simulink model "model20Drones"  (R2022a)
settings: Solver=FixedStepAuto  StartTime=0.0  StopTime=inf  FixedStep=1  RelTol=1e-3
values from neighbouring files (symbols this model uses):
  droneCount = 3    [workspace.mat]
  map = [0 0 0 0 0 0 0 0 0 0 99 99 ... (400 elements, 20x20)]    [workspace.mat]
libraries: drone x20
settings Model: Creator=JadKHaddad  LastModifiedBy=JadKHaddad

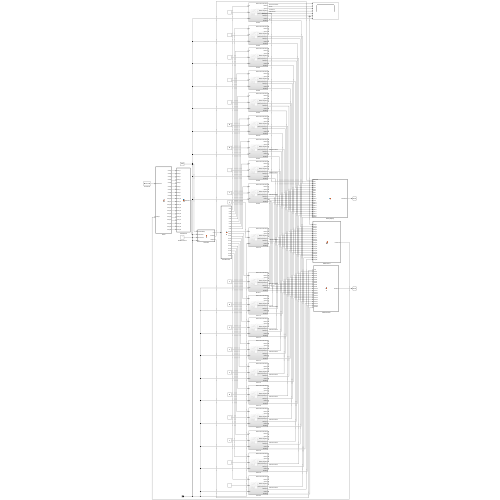
[thumbnail: Simulink's stored preview of the top-level diagram]
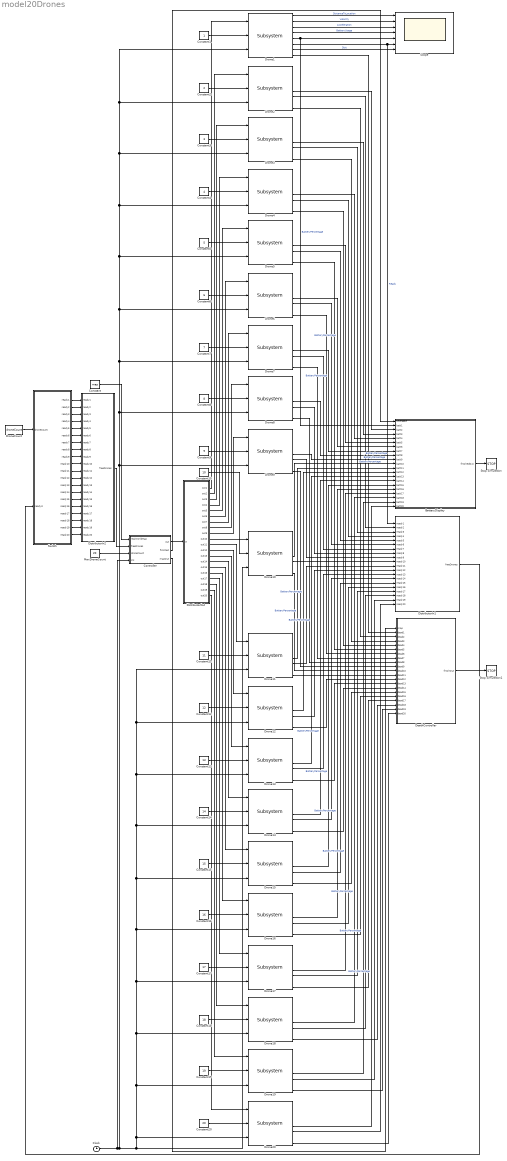
== system model20Drones ==
  BatteryDisplay : MATLAB Function  TreatAsAtomicUnit=on
  Clock : Clock
  Constant : Constant  Value=map  VectorParams1D=off
  Constant1 : Constant
  Constant10 : Constant  Value=10
  Constant11 : Constant  Value=11
  Constant12 : Constant  Value=12
  Constant13 : Constant  Value=13
  Constant14 : Constant  Value=14
  Constant15 : Constant  Value=15
  Constant16 : Constant  Value=16
  Constant17 : Constant  Value=17
  Constant18 : Constant  Value=18
  Constant19 : Constant  Value=19
  Constant2 : Constant  Value=2
  Constant20 : Constant  Value=20
  Constant3 : Constant  Value=3
  Constant4 : Constant  Value=4
  Constant5 : Constant  Value=5
  Constant6 : Constant  Value=6
  Constant7 : Constant  Value=7
  Constant8 : Constant  Value=8
  Constant9 : Constant  Value=9
  Controller : MATLAB Function  TreatAsAtomicUnit=on
  DeathController : MATLAB Function  TreatAsAtomicUnit=on
  DistributorIn1 : MATLAB Function  TreatAsAtomicUnit=on
  DistributorIn2 : MATLAB Function  TreatAsAtomicUnit=on
  DistributorOut : MATLAB Function  TreatAsAtomicUnit=on
  Drone{1..5,7..20} (19 alike) : drone/Subsystem  SystemSampleTime=-1  VariantActivationTime=update diagram  Latency=0  AutoFrameSizeCalculation=off
  "Drone6 " : drone/Subsystem  SystemSampleTime=-1  VariantActivationTime=update diagram  Latency=0  AutoFrameSizeCalculation=off
  DroneCount : Constant  Value=droneCount
  MaxDroneCount : Constant  Value=20
  Scope : Scope  NumInputPorts=7
  Stop Simulation : Stop
  Stop Simulation1 : Stop
  Switch : MATLAB Function  TreatAsAtomicUnit=on
  wires:
  Drone2/5 -> BatteryDisplay/3(batt2)
  DistributorOut/15(out15) -> Drone15/1
  Drone20/5 -> BatteryDisplay/21(batt20)  "BatteryPercentage"
  Switch/18(ready18) -> DistributorIn2/18(ready18)
  Drone19/5 -> BatteryDisplay/20(batt19)  "BatteryPercentage"
  Drone19/6 -> DistributorIn1/19(ready19)
  Constant13/1 -> Drone13/2
  Drone14/8 -> DeathController/15(dead14)
  DistributorOut/20(out20) -> Drone20/1
  Drone13/6 -> DistributorIn1/13(ready13)
  Clock/1 -> Drone12/3, Drone11/3, Drone13/3, Drone14/3, Drone15/3, Drone16/3, Drone17/3, Drone18/3, Drone19/3, Drone20/3, Drone10/3, Drone2/3, Drone1/3, Drone3/3, Drone4/3, Drone5/3, "Drone6 "/3, Drone7/3, Drone8/3, Drone9/3, Controller/4(clk)
  DistributorOut/19(out19) -> Drone19/1
  Drone17/8 -> DeathController/18(dead17)
  Drone20/6 -> DistributorIn1/20(ready20)
  Constant17/1 -> Drone17/2
  Switch/8(ready8) -> DistributorIn2/8(ready8)
  Drone19/8 -> DeathController/20(dead19)
  Drone11/5 -> BatteryDisplay/12(batt11)  "BatteryPercentage"
  Drone20/8 -> DeathController/21(dead20)
  Constant20/1 -> Drone20/2
  Switch/17(ready17) -> DistributorIn2/17(ready17)
  Drone15/5 -> BatteryDisplay/16(batt15)  "BatteryPercentage"
  Constant19/1 -> Drone19/2
  Drone18/5 -> BatteryDisplay/19(batt18)  "BatteryPercentage"
  Drone18/6 -> DistributorIn1/18(ready18)
  DistributorOut/5(out5) -> Drone5/1
  Drone18/8 -> DeathController/19(dead18)
  DistributorOut/18(out18) -> Drone18/1
  Drone11/6 -> DistributorIn1/11(ready11)
  Constant9/1 -> Drone9/2
  DistributorOut/17(out17) -> Drone17/1
  Constant18/1 -> Drone18/2
  Drone17/5 -> BatteryDisplay/18(batt17)  "BatteryPercentage"
  Drone17/6 -> DistributorIn1/17(ready17)
  Drone16/5 -> BatteryDisplay/17(batt16)  "BatteryPercentage"
  Drone16/8 -> DeathController/17(dead16)
  Drone16/6 -> DistributorIn1/16(ready16)
  Switch/12(ready12) -> DistributorIn2/12(ready12)
  DistributorOut/16(out16) -> Drone16/1
  Constant16/1 -> Drone16/2
  Drone15/6 -> DistributorIn1/15(ready15)
  Drone15/8 -> DeathController/16(dead15)
  Constant15/1 -> Drone15/2
  Switch/15(ready15) -> DistributorIn2/15(ready15)
  Drone14/6 -> DistributorIn1/14(ready14)
  Drone14/5 -> BatteryDisplay/15(batt14)  "BatteryPercentage"
  "Drone6 "/5 -> BatteryDisplay/7(batt6)  "BatteryPercentage"
  DistributorOut/14(out14) -> Drone14/1
  Constant14/1 -> Drone14/2
  Drone13/8 -> DeathController/14(dead13)
  Switch/5(ready5) -> DistributorIn2/5(ready5)
  Constant10/1 -> Drone10/2
  Switch/11(ready11) -> DistributorIn2/11(ready11)
  Switch/1(ready1) -> DistributorIn2/1(ready1)
  Drone13/5 -> BatteryDisplay/14(batt13)  "BatteryPercentage"
  DistributorOut/13(out13) -> Drone13/1
  Drone12/6 -> DistributorIn1/12(ready12)
  Drone12/8 -> DeathController/13(dead12)
  Drone12/5 -> BatteryDisplay/13(batt12)  "BatteryPercentage"
  DistributorOut/12(out12) -> Drone12/1
  Drone11/8 -> DeathController/12(dead11)
  Drone2/8 -> DeathController/3(dead2)
  Constant12/1 -> Drone12/2
  Constant11/1 -> Drone11/2
  DistributorOut/11(out11) -> Drone11/1
  Switch/20(ready20) -> DistributorIn2/20(ready20)
  Drone1/7 -> Scope/7  "Dist"
  Switch/19(ready19) -> DistributorIn2/19(ready19)
  Switch/16(ready16) -> DistributorIn2/16(ready16)
  Switch/14(ready14) -> DistributorIn2/14(ready14)
  Switch/13(ready13) -> DistributorIn2/13(ready13)
  Drone3/5 -> BatteryDisplay/4(batt3)
  Switch/4(ready4) -> DistributorIn2/4(ready4)
  Switch/3(ready3) -> DistributorIn2/3(ready3)
  DistributorOut/1(out1) -> Drone1/1
  DroneCount/1 -> Switch/1(droneCount)
  DistributorOut/3(out3) -> Drone3/1
  Drone2/6 -> DistributorIn1/2(ready2)
  Controller/2(finished) -> BatteryDisplay/1(finishedIn)
  DistributorOut/9(out9) -> Drone9/1
  Controller/3(mapOut) -> DeathController/1(map)
  DistributorIn2/1(freeDrones) -> Controller/2(freeDrones)
  Drone1/2 -> Scope/2  "Velocity"
  DistributorIn1/1(freeDrones) -> Switch/2(readyIn)
  Constant1/1 -> Drone1/2
  BatteryDisplay/1(finishedOut) -> Stop Simulation/1
  Constant3/1 -> Drone3/2
  Drone1/8 -> DeathController/2(dead1)
  Drone1/4 -> Scope/4  "BatteryUsage"
  Controller/1(out) -> DistributorOut/1(in)
  DistributorOut/4(out4) -> Drone4/1
  DistributorOut/2(out2) -> Drone2/1
  Constant5/1 -> Drone5/2
  Drone4/5 -> BatteryDisplay/5(batt4)
  Drone1/1 -> Scope/1  "DistanceToLocation"
  Drone5/5 -> BatteryDisplay/6(batt5)
  Switch/2(ready2) -> DistributorIn2/2(ready2)
  Constant/1 -> Controller/1(realWorldMap)
  Drone3/8 -> DeathController/4(dead3)
  Constant2/1 -> Drone2/2
  Drone4/6 -> DistributorIn1/4(ready4)
  DeathController/1(finishOut) -> Stop Simulation1/1
  Switch/6(ready6) -> DistributorIn2/6(ready6)
  Switch/7(ready7) -> DistributorIn2/7(ready7)
  Switch/9(ready9) -> DistributorIn2/9(ready9)
  Constant8/1 -> Drone8/2
  Constant6/1 -> "Drone6 "/2
  DistributorOut/6(out6) -> "Drone6 "/1
  DistributorOut/7(out7) -> Drone7/1
  Drone1/3 -> Scope/3  "Acceleration"
  DistributorOut/8(out8) -> Drone8/1
  DistributorOut/10(out10) -> Drone10/1
  MaxDroneCount/1 -> Controller/3(droneCount)
  "Drone6 "/8 -> DeathController/7(dead6)
  Drone7/8 -> DeathController/8(dead7)
  Drone8/8 -> DeathController/9(dead8)
  Switch/10(ready10) -> DistributorIn2/10(ready10)
  Drone9/8 -> DeathController/10(dead9)
  Drone5/8 -> DeathController/6(dead5)
  Drone10/8 -> DeathController/11(dead10)
  Drone7/6 -> DistributorIn1/7(ready7)
  Drone9/6 -> DistributorIn1/9(ready9)
  Drone3/6 -> DistributorIn1/3(ready3)
  Constant4/1 -> Drone4/2
  Drone8/6 -> DistributorIn1/8(ready8)
  Drone7/5 -> BatteryDisplay/8(batt7)  "BatteryPercentage"
  Drone5/6 -> DistributorIn1/5(ready5)
  Drone8/5 -> BatteryDisplay/9(batt8)  "BatteryPercentage"
  "Drone6 "/6 -> DistributorIn1/6(ready6)
  Constant7/1 -> Drone7/2
  Drone9/5 -> BatteryDisplay/10(batt9)  "BatteryPercentage"
  Drone10/6 -> DistributorIn1/10(ready10)
  Drone4/8 -> DeathController/5(dead4)
  Drone10/5 -> BatteryDisplay/11(batt10)  "BatteryPercentage"
  Drone1/6 -> Scope/6, DistributorIn1/1(ready1)  "Ready"
  Drone1/5 -> BatteryDisplay/2(batt1), Scope/5  "BatteryPercentage"

== matlab function model20Drones/DeathController ==
  data: map input; finishOut output; dead1 input; dead2 input; dead3 input; dead4 input; dead5 input; dead6 input; dead7 input; dead8 input; dead9 input; dead10 input; dead11 input; dead12 input; dead13 input; dead14 input; dead15 input; dead16 input; dead17 input; dead18 input; dead19 input; dead20 input
function finishOut = fcn(map, dead1, dead2, dead3, dead4, dead5, dead6, dead7, dead8, dead9, dead10, dead11, dead12, dead13, dead14, dead15, dead16, dead17, dead18, dead19, dead20)
    %stops the simulation if all drones are dead
    allDead = 0;
    if dead1 == 1 && dead2 == 1 && dead3 == 1 && dead4 == 1 && dead5 == 1 && dead6 == 1 && dead7 == 1 && dead8 == 1 && dead9 == 1 && dead10 == 1 && dead11 == 1 && dead12 == 1 && dead13 == 1 && dead14 == 1 && dead15 == 1 && dead16 == 1 && dead17 == 1 && dead18 == 1 && dead19 == 1 && dead20 == 1
        allDead = 1;
    end
    if allDead == 1
        fprintf("All drones died. Terminating...\n\nMap:\n");
        disp(map);
    end
    finishOut = allDead;
end

== matlab function model20Drones/Switch ==
  data: droneCount input; ready1 output; readyIn input; ready2 output; ready3 output; ready4 output; ready5 output; ready6 output; ready7 output; ready8 output; ready9 output; ready10 output; ready11 output; ready12 output; ready13 output; ready14 output; ready15 output; ready16 output; ready17 output; ready18 output; ready19 output; ready20 output
function [ready1, ready2, ready3, ready4, ready5, ready6, ready7, ready8, ready9, ready10, ready11, ready12, ready13, ready14, ready15, ready16, ready17, ready18, ready19, ready20] = fcn(droneCount, readyIn)
    %configures the desired drone count
    out = zeros(20);
    i = 1;
    while i <= droneCount
        out(i) = readyIn(i);
        i = i +1;
    end
    
    ready1 = out(1);
    ready2 = out(2);
    ready3 = out(3);
    ready4 = out(4);
    ready5 = out(5);
    ready6 = out(6);
    ready7 = out(7);
    ready8 = out(8);
    ready9 = out(9);
    ready10 = out(10);
    ready11 = out(11);
    ready12 = out(12);
    ready13 = out(13);
    ready14 = out(14);
    ready15 = out(15);
    ready16 = out(16);
    ready17 = out(17);
    ready18 = out(18);
    ready19 = out(19);
    ready20 = out(20);
    
end

== matlab function model20Drones/DistributorIn1 ==
  data: ready1 input; freeDrones output; ready2 input; ready3 input; ready4 input; ready5 input; ready6 input; ready7 input; ready8 input; ready9 input; ready10 input; ready11 input; ready12 input; ready13 input; ready14 input; ready15 input; ready16 input; ready17 input; ready18 input; ready19 input; ready20 input
function freeDrones = fcn(ready1, ready2, ready3, ready4, ready5, ready6, ready7, ready8, ready9, ready10, ready11, ready12, ready13, ready14, ready15, ready16, ready17, ready18, ready19, ready20)
    %collects the "ready signal" from all drones to a single port
    freeDrones = [ready1 ready2 ready3 ready4 ready5 ready6 ready7 ready8 ready9 ready10 ready11 ready12 ready13 ready14 ready15 ready16 ready17 ready18 ready19 ready20];
end

== matlab function model20Drones/Controller ==
  settings: updateMethod=DISCRETE
  data: realWorldMap input; out output; finished output; freeDrones input; droneCount input; mapOut output; clk input
function [out, finished, mapOut] = fcn(realWorldMap, freeDrones, droneCount, clk)
    persistent index
    persistent indexLimit
    persistent path
    persistent lastXY
    persistent workingDronesCount
    persistent cameBackDronesCount
    persistent map
    persistent workingDrones
    persistent inTermMode
    
    %init persistent values
    if isempty(inTermMode)
        inTermMode = 0;
    end
    if isempty(workingDrones)
        workingDrones = zeros(droneCount);
    end
    if isempty(workingDronesCount)
        workingDronesCount = 0;
    end
    if isempty(cameBackDronesCount)
        cameBackDronesCount = 0;
    end
    if isempty(index)
        index = 1;
    end
    if isempty(indexLimit)
        indexLimit = 2;
    end
    if isempty(path)
        path = ones(length(realWorldMap)*length(realWorldMap),2);
    end
    if isempty(lastXY)
        lastXY = ones(droneCount, 2);
        lastXY = -1 * lastXY;
    end
    if isempty(map)
        map = zeros(length(realWorldMap), length(realWorldMap));
    end
    
    %returns the index of a drone with the minimal distance to a given position on the map - returns -1 if there is no free path
    function indexDist = getIndexAndDistOfAFreeDrone(dest)
        DIndex = -1;
        minDist = -1;
        i = 1;
        while(i <= droneCount)
            if(freeDrones(i) == 1)
                source = lastXY(i,:);
                if source(1) == -2
                    i = i + 1;
                    continue
                end
                if(source(1) == -1)
                    source(1) = 1;
                end
                if(source(2) == -1)
                    source(2) = 1;
                end
                dist = minDistanceSimulink(map, source(1), source(2), dest(1), dest(2));
                if(minDist == -1 && dist ~= -1) || (minDist ~= -1 && dist ~= -1 && dist < minDist)
                    minDist = dist;
                    DIndex = i;
                end
            end
            i = i + 1;
        end
        indexDist = [DIndex minDist];
    end

    finished = 0;
    mapOut = map;
    
    %init out port
    out = ones(20, 4); % = [x y dist vld];
    i = 1;
    while (i <= droneCount)
       out(i,:) = [1 1 -1 0];
       i = i + 1;
    end

    %sink - acts like a sink - receives signals from the drones and updates the locations that can be discovered
    if cameBackDronesCount >= droneCount
        %if all drones came back - print results and terminate
        finished = 1;
        fprintf("[%d]: All drones came back. Terminating...\n\nMap:\n", int32(clk));
        disp(map);
        return
    end
    %check if a drone has finished it's trip
    i = 1;
    while i <= droneCount
        x = lastXY(i, 1);
        y = lastXY(i, 2);
        droneIsFree = freeDrones(1, i);
        if droneIsFree == 1 && x == -2 %drone came back to start location
            cameBackDronesCount = cameBackDronesCount + 1;
            fprintf("[%d]: Drone [%d] came back\n", int32(clk), int8(i));
            lastXY(i,:) = [-3 -3];
            i = i + 1;
            continue
        end
        if droneIsFree == 1 && x ~= -1 && x ~= -2 && x ~= -3 && workingDrones(i) == 1 %drone has finished a trip
            fprintf("[%d]: Drone [%d] is now ready\n", int32(clk), int8(i));
            workingDrones(i) = 0;
            workingDronesCount = workingDronesCount - 1;
            %mark current drone location as dynamically blocked
            map(x,y) = 3;
            %update path - add new locations to the path that can be
            %discovered - based on the new discovered location
            if realWorldMap(x,y) == 0
                if x + 1 <= length(realWorldMap) && map(x + 1, y) == 0
                    if realWorldMap(x + 1, y) == 0
                        newRow = [x+1 y];
                        map(x+1,y) = -1;
                        path(indexLimit,:) = newRow;
                        indexLimit = indexLimit + 1;
                    else
                        map(x+1,y) = 99;
                    end
                end
                
                if y + 1 <= length(realWorldMap) && map(x, y + 1) == 0
                    if realWorldMap(x, y + 1) == 0
                        newRow = [x y+1];
                        map(x,y+1) = -1;
                        path(indexLimit,:) = newRow;
                        indexLimit = indexLimit + 1;
                    else
                        map(x, y + 1) = 99;
                    end
                end
                
                if x - 1 >= 1 && map(x - 1, y) == 0 
                    if realWorldMap(x - 1, y) == 0 
                        newRow = [x-1 y];
                        map(x-1,y) = -1;
                        path(indexLimit,:) = newRow;
                        indexLimit = indexLimit + 1;
                    else
                        map(x - 1, y) = 99;
                    end
                end
                
                if y - 1 >= 1 && map(x, y-1) == 0
                    if realWorldMap(x, y-1) == 0
                        newRow = [x y-1];
                        map(x,y-1) = -1;
                        path(indexLimit,:) = newRow;
                        indexLimit = indexLimit + 1;
                    else
                        map(x, y-1) = 99;
                    end
                end
            end
            j = index;
            fprintf("[%d]: Next free positions: ", int32(clk));
            while j < indexLimit
                fprintf("(%d, %d) ", int8(path(j,1)), int8(path(j,2)));
                j = j + 1;
            end
            fprintf("\n");
        end
        i = i + 1;
    end
    %end of sink

    %source 
    %check if all free locations have been checked
    if index >= indexLimit
        if workingDronesCount == 0
            %if there is not a single drone working - call drones back to start location - exit the source
            %if there is a working drone - wait
            if inTermMode == 0
                fprintf("[%d]: Entering termination mode\n", int32(clk));
                inTermMode = 1;
            end
            %call drones to start location
            droneIndex = 1;
            while droneIndex <= droneCount
                droneLocation = lastXY(droneIndex,:);
                if droneLocation(1) == -1 %drone is still at start location - does not happen in the 3 given scenarios
                    fprintf("[%d]: Drone [%d] is already at start location\n", int32(clk), int8(droneIndex));
                    lastXY(droneIndex, :) = [-3 -3];
                    cameBackDronesCount = cameBackDronesCount + 1;
                    droneIndex = droneIndex + 1;
                    continue
                end
                %if a drone already came back or is on the was - ignore
                if droneLocation(1) == -3 || droneLocation(1) == -2
                    droneIndex = droneIndex + 1;
                    continue
                end
                droneIsFree = freeDrones(1, droneIndex);
                %calling a drone to the start location
                if droneIsFree == 1
                    dist = minDistanceSimulink(map, droneLocation(1), droneLocation(2), 1, 1);
                    out(droneIndex,1) = -2;
                    out(droneIndex,2) = -2;
                    out(droneIndex,3) = dist;
                    out(droneIndex,4) = 1;
                    fprintf("[%d]: Calling drone [%d] back from(%d, %d) with distance [%d]\n", int32(clk), int8(droneIndex), int8(lastXY(droneIndex,1)), int8(lastXY(droneIndex,2)), int8(dist));
                    %mark drone's last location as discovered
                    map(droneLocation(1), droneLocation(2)) = 1;
                    %set the new drone's location - (-2, -2): on the way
                    %back
                    lastXY(droneIndex,:) = [-2 -2];
                end
                droneIndex = droneIndex + 1;
            end
        end
    %select next location to be discovered - find drone with minimum distance
    else
        dest = path(index,:);
        indexDist = getIndexAndDistOfAFreeDrone(dest);
        droneIndex = indexDist(1);
        dist = indexDist(2);
        %if a free path exists - send the drone
        if droneIndex > -1 && dist > -1
            out(droneIndex,1) = dest(1);
            out(droneIndex,2) = dest(2);
            out(droneIndex,3) = dist;
            out(droneIndex,4) = 1;
            fprintf("[%d]: Sending drone [%d] from (%d, %d) to (%d, %d) with distance [%d]\n", int32(clk), int8(droneIndex), int8(lastXY(droneIndex,1)), int8(lastXY(droneIndex,2)), int8(dest(1)), int8(dest(2)), int8(dist));
            workingDronesCount = workingDronesCount + 1;
            workingDrones(droneIndex) = 1;
            if lastXY(droneIndex,1) ~= -1
                if map(lastXY(droneIndex,1), lastXY(droneIndex,2)) == 3
                    map(lastXY(droneIndex,1), lastXY(droneIndex,2)) = 1;
                end
            end
            %mark destination "to be discovered"
            map(dest(1),dest(2)) = 2;
            %save drone's new location
            lastXY(droneIndex,:) = dest;
            index = index + 1;
        end
    end
    %end of source
end

== matlab function model20Drones/DistributorOut ==
  data: in input; out1 output; out2 output; out3 output; out4 output; out5 output; out6 output; out7 output; out8 output; out9 output; out10 output; out11 output; out12 output; out13 output; out14 output; out15 output; out16 output; out17 output; out18 output; out19 output; out20 output
function [out1, out2, out3, out4, out5, out6, out7, out8, out9, out10, out11, out12, out13, out14, out15, out16, out17, out18, out19, out20] = fcn(in)
    %distributes the out signal from the controller to the drones
    out1 = [1 1 -1 0];
    out2 = [1 1 -1 0];    
    out3 = [1 1 -1 0];
    out4 = [1 1 -1 0];    
    out5 = [1 1 -1 0];
    out6 = [1 1 -1 0];
    out7 = [1 1 -1 0];    
    out8 = [1 1 -1 0];
    out9 = [1 1 -1 0];    
    out10 = [1 1 -1 0];
    out11 = [1 1 -1 0];
    out12 = [1 1 -1 0];    
    out13 = [1 1 -1 0];
    out14 = [1 1 -1 0];    
    out15 = [1 1 -1 0];
    out16 = [1 1 -1 0];
    out17 = [1 1 -1 0];    
    out18 = [1 1 -1 0];
    out19 = [1 1 -1 0];    
    out20 = [1 1 -1 0];
    
    out1 = in(1,:);
    out2 = in(2,:);
    out3 = in(3,:);
    out4 = in(4,:);
    out5 = in(5,:);
    out6 = in(6,:);
    out7 = in(7,:);
    out8 = in(8,:);
    out9 = in(9,:);
    out10 = in(10,:);
    out11 = in(11,:);
    out12 = in(12,:);
    out13 = in(13,:);
    out14 = in(14,:);
    out15 = in(15,:);
    out16 = in(16,:);
    out17 = in(17,:);
    out18 = in(18,:);
    out19 = in(19,:);
    out20 = in(20,:);
end

== matlab function model20Drones/DistributorIn2 ==
  data: ready1 input; freeDrones output; ready2 input; ready3 input; ready4 input; ready5 input; ready6 input; ready7 input; ready8 input; ready9 input; ready10 input; ready11 input; ready12 input; ready13 input; ready14 input; ready15 input; ready16 input; ready17 input; ready18 input; ready19 input; ready20 input
function freeDrones = fcn(ready1, ready2, ready3, ready4, ready5, ready6, ready7, ready8, ready9, ready10, ready11, ready12, ready13, ready14, ready15, ready16, ready17, ready18, ready19, ready20)
    %collects the "ready signal" from all drones to a single port
    freeDrones = [ready1 ready2 ready3 ready4 ready5 ready6 ready7 ready8 ready9 ready10 ready11 ready12 ready13 ready14 ready15 ready16 ready17 ready18 ready19 ready20];
end

== matlab function model20Drones/BatteryDisplay ==
  data: finishedIn input; finishedOut output; batt1 input; batt2 input; batt3 input; batt4 input; batt5 input; batt6 input; batt7 input; batt8 input; batt9 input; batt10 input; batt11 input; batt12 input; batt13 input; batt14 input; batt15 input; batt16 input; batt17 input; batt18 input; batt19 input; batt20 input
function finishedOut = fcn(finishedIn, batt1, batt2, batt3, batt4, batt5, batt6, batt7, batt8, batt9, batt10, batt11, batt12, batt13, batt14, batt15, batt16, batt17, batt18, batt19, batt20)
    %displays battery percentage of all drones and terminates the
    %simulation
    finishedOut = finishedIn;
    if finishedIn == 1
        fprintf("\n\n");
        fprintf("Drone [1] battery capacity: [%f%%]\n", batt1*100);
        fprintf("Drone [2] battery capacity: [%f%%]\n", batt2*100);
        fprintf("Drone [3] battery capacity: [%f%%]\n", batt3*100);
        fprintf("Drone [4] battery capacity: [%f%%]\n", batt4*100);
        fprintf("Drone [5] battery capacity: [%f%%]\n", batt5*100);
        fprintf("Drone [6] battery capacity: [%f%%]\n", batt6*100);
        fprintf("Drone [7] battery capacity: [%f%%]\n", batt7*100);
        fprintf("Drone [8] battery capacity: [%f%%]\n", batt8*100);
        fprintf("Drone [9] battery capacity: [%f%%]\n", batt9*100);
        fprintf("Drone [10] battery capacity: [%f%%]\n", batt10*100);
        fprintf("Drone [11] battery capacity: [%f%%]\n", batt11*100);
        fprintf("Drone [12] battery capacity: [%f%%]\n", batt12*100);
        fprintf("Drone [13] battery capacity: [%f%%]\n", batt13*100);
        fprintf("Drone [14] battery capacity: [%f%%]\n", batt14*100);
        fprintf("Drone [15] battery capacity: [%f%%]\n", batt15*100);
        fprintf("Drone [16] battery capacity: [%f%%]\n", batt16*100);
        fprintf("Drone [17] battery capacity: [%f%%]\n", batt17*100);
        fprintf("Drone [18] battery capacity: [%f%%]\n", batt18*100);
        fprintf("Drone [19] battery capacity: [%f%%]\n", batt19*100);
        fprintf("Drone [20] battery capacity: [%f%%]\n", batt20*100);
    end
end
